simulink model "FinalProject"  (R2025b)
settings: Solver=ode3  StartTime=0.0  StopTime=1  RelTol=1e-3
libraries: spsMosfetLib x12, simulink x9, spsDCVoltageSourceLib x4, spsCurrentMeasurementLib x1, spsSeriesRLCBranchLib x1, spsVoltageMeasurementLib x1, sps_lib x1
settings Model: Creator=RGUKT  LastModifiedBy=RGUKT

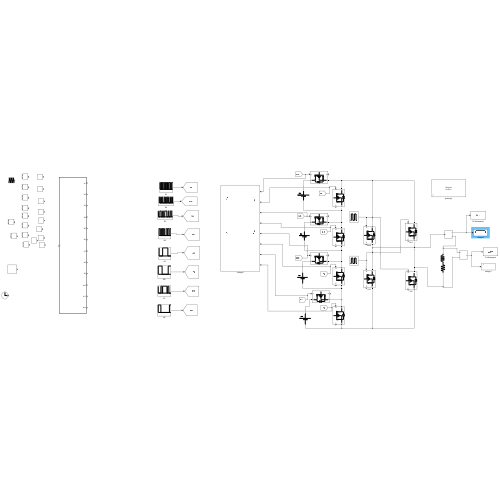
[thumbnail: Simulink's stored preview of the top-level diagram]
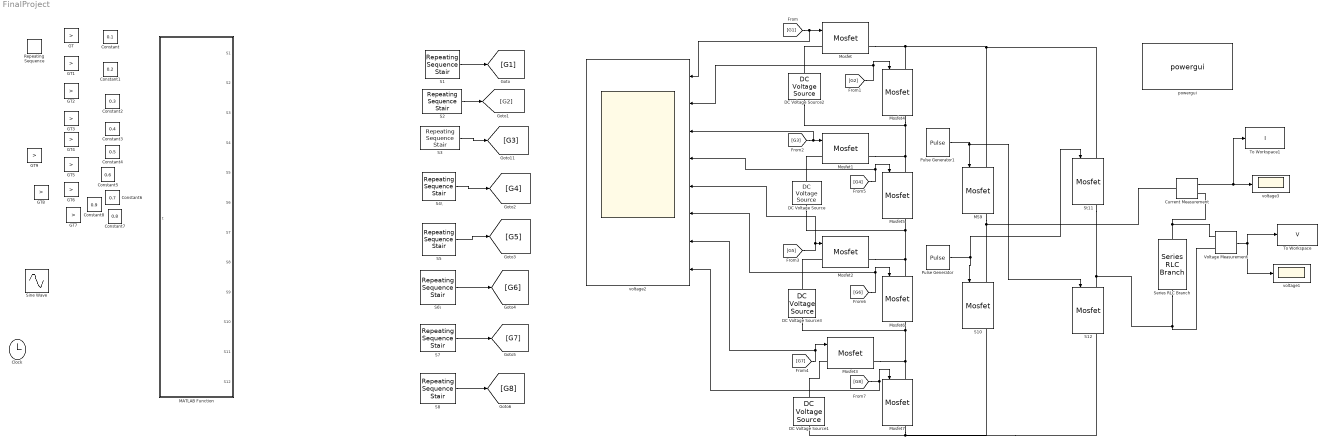
== system FinalProject ==
  Clock : Clock
  Constant : Constant  Value=0.1
  Constant1 : Constant  Value=0.2
  Constant2 : Constant  Value=0.3
  Constant3 : Constant  Value=0.4
  Constant4 : Constant  Value=0.5
  Constant5 : Constant  Value=0.6
  Constant6 : Constant  Value=0.7
  Constant7 : Constant  Value=0.8
  Constant8 : Constant  Value=0.9
  Current Measurement : spsCurrentMeasurementLib/Current Measurement  PhasorSimulation=off  OutputType=Complex  PSBequivalent=0
  DC Voltage Source : spsDCVoltageSourceLib/DC Voltage Source  Amplitude=20  Measurements=None
  DC Voltage Source1 : spsDCVoltageSourceLib/DC Voltage Source  Amplitude=40  Measurements=None
  DC Voltage Source2 : spsDCVoltageSourceLib/DC Voltage Source  Amplitude=10  Measurements=None
  DC Voltage Source3 : spsDCVoltageSourceLib/DC Voltage Source  Amplitude=30  Measurements=None
  GT{,1..9} (10 alike) : RelationalOperator  Operator=>  OutDataTypeStr=boolean  RndMeth=Simplest  InputSameDT=off
  MATLAB Function : MATLAB Function  TreatAsAtomicUnit=on
  MS9 : spsMosfetLib/Mosfet  Ron=0.1  Lon=0  Rd=0.01  Vfd=0  IC=0  Rs=1e5  Cs=inf  Measurements=on
  Mosfet{,1..7} (8 alike) : spsMosfetLib/Mosfet  Ron=0.1  Lon=0  Rd=0.01  Vfd=0  IC=0  Rs=1e5  Cs=inf  Measurements=on
  Pulse Generator : DiscretePulseGenerator  PulseType=Time based  Period=0.02  PulseWidth=50  PhaseDelay=0.01
  Pulse Generator1 : DiscretePulseGenerator  PulseType=Time based  Period=0.02  PulseWidth=50
  Repeating Sequence : simulink/Sources/Repeating Sequence  rep_seq_t=[0 0.01 0.02]  rep_seq_y=[0 1 0]
  S1 : simulink/Sources/Repeating Sequence Stair  OutValues=[0 1 0 1 0 1 1 0 1 0 1 0 1 0 1 1 0 1 0 1].'  tsamp=0.0005  OutMin=[]  OutMax=[]  OutDataTypeStr=double  OutputDataTypeScalingMode=double  OutDataType=fixdt(0,8)  ConRadixGroup=Best Precision: Vector-wise  OutScaling=2^-12
  S10 : spsMosfetLib/Mosfet  Ron=0.1  Lon=0  Rd=0.01  Vfd=0  IC=0  Rs=1e5  Cs=inf  Measurements=on
  S12 : spsMosfetLib/Mosfet  Ron=0.1  Lon=0  Rd=0.01  Vfd=0  IC=0  Rs=1e5  Cs=inf  Measurements=on
  S2 : simulink/Sources/Repeating Sequence Stair  OutValues=[1 0 1 0 1 0 0 1 0 1 0 1 0 1 0 0 1 0 1 0].'  tsamp=0.0005  OutMin=[]  OutMax=[]  OutDataTypeStr=double  OutputDataTypeScalingMode=double  OutDataType=fixdt(0,8)  ConRadixGroup=Best Precision: Vector-wise  OutScaling=2^-12
  S3 : simulink/Sources/Repeating Sequence Stair  OutValues=[0 0 1 1 0 0 1 0 0 1 1 1 0 0 1 0 0 1 1 0].'  tsamp=0.0005  OutMin=[]  OutMax=[]  OutDataTypeStr=double  OutputDataTypeScalingMode=double  OutDataType=fixdt(0,8)  ConRadixGroup=Best Precision: Vector-wise  OutScaling=2^-12
  S4\ : simulink/Sources/Repeating Sequence Stair  OutValues=[1 1 0 0 1 1 0 1 1 0 0 0 1 1 0 1 1 0 0 1].'  tsamp=0.0005  OutMin=[]  OutMax=[]  OutDataTypeStr=double  OutputDataTypeScalingMode=double  OutDataType=fixdt(0,8)  ConRadixGroup=Best Precision: Vector-wise  OutScaling=2^-12
  S5 : simulink/Sources/Repeating Sequence Stair  OutValues=[0 0 0 0 0 0 1 1 1 1 1 1 1 1 1 0 0 0 0 0].'  tsamp=0.0005  OutMin=[]  OutMax=[]  OutDataTypeStr=double  OutputDataTypeScalingMode=double  OutDataType=fixdt(0,8)  ConRadixGroup=Best Precision: Vector-wise  OutScaling=2^-12
  S6\ : simulink/Sources/Repeating Sequence Stair  OutValues=[1 1 1 1 1 1 0 0 0 0 0 0 0 0 0 0 1 1 1 1].'  tsamp=0.0005  OutMin=[]  OutMax=[]  OutDataTypeStr=double  OutputDataTypeScalingMode=double  OutDataType=fixdt(0,8)  ConRadixGroup=Best Precision: Vector-wise  OutScaling=2^-12
  S7 : simulink/Sources/Repeating Sequence Stair  OutValues=[0 0 0 0 1 1 0 1 1 1 1 1 1 1 0 1 1 0 0 0].'  tsamp=0.0005  OutMin=[]  OutMax=[]  OutDataTypeStr=double  OutputDataTypeScalingMode=double  OutDataType=fixdt(0,8)  ConRadixGroup=Best Precision: Vector-wise  OutScaling=2^-12
  S8 : simulink/Sources/Repeating Sequence Stair  OutValues=[1 1 1 1 0 0 0 0 0 0 0 0 0 0 0 0 0 0 1 1].'  tsamp=0.0005  OutMin=[]  OutMax=[]  OutDataTypeStr=double  OutputDataTypeScalingMode=double  OutDataType=fixdt(0,8)  ConRadixGroup=Best Precision: Vector-wise  OutScaling=2^-12
  Series RLC Branch : spsSeriesRLCBranchLib/Series RLC Branch  LConnTagsString=__new0  RConnTagsString=__new0  BranchType=RL  Resistance=10  Inductance=0.007  SetiL0=off  InitialCurrent=0  Capacitance=1e-6  Setx0=off  InitialVoltage=0  Measurements=None
  Sine Wave : Sin  Frequency=314.15  SampleTime=0
  St11 : spsMosfetLib/Mosfet  Ron=0.1  Lon=0  Rd=0.01  Vfd=0  IC=0  Rs=1e5  Cs=inf  Measurements=on
  To Workspace : ToWorkspace  VariableName=V  SaveFormat=Structure With Time  SampleTime=-1
      settings: Save2DSignal=2-D array (concatenate along first dimension)
  To Workspace1 : ToWorkspace  VariableName=I  SaveFormat=Structure With Time  SampleTime=-1
      settings: Save2DSignal=2-D array (concatenate along first dimension)
  Voltage Measurement : spsVoltageMeasurementLib/Voltage Measurement  PhasorSimulation=off  OutputType=Complex  PSBequivalent=0
  powergui : sps_lib/powergui  Priority=1  SimulationMode=Discrete  SampleTime=5e-06  frequency=60  Iterations=50  frequencyindice=0  Pbase=100e6  ErrMax=1e-4  UnitsV=kV  UnitsW=MW  buscounter=0  FunctionMessages=off  echomessages=off  EnableUseOfTLC=off  CurrentSourceSwitches=off  DisableSnubberDevices=off  DisableRonSwitches=off  DisableVfSwitches=off  DisplayEquations=off  AutomaticDiscreteSolvers=off  SolverType=Tustin/Backward Euler (TBE)  Interpol=off  ExternalGateDelay=off  methode=off  Ts=100  x0status=blocks  SPID=on  SwTol=0  HookPort=off  NonlinearTolerance=1e-4  nMaxIteration=100  ContinueOnMaxIteration=off  RestoreLinks=warning  ResistiveCurrentMeasurement=off  Frange=[0:2:500]  Ylog=off  Xlog=on  ShowGrid=off  save=off  variable=ZData  structure=0  ZoomFFT=off  StartTime=0.0  cycles=1  DisplayStyle=1  fundamental=60  FreqAxis=off  MaxFrequency=1000  frequencyindicesteady=1  RmsSteady=1  display=off
  voltage1 : Scope
      settings: ActiveDisplayYMinimum=-117.92329789248066  ActiveDisplayYMaximum=117.9232978938367
  voltage2 : Scope  NumInputPorts=8
      settings: ActiveDisplayYMinimum=-0.12499999999999997  ActiveDisplayYMaximum=1.125  DataLoggingVariableName=ScopeData2
  voltage3 : Scope
      settings: ActiveDisplayYMinimum=-11.792329789248956  ActiveDisplayYMaximum=11.7923297893823
  wires:
  Voltage Measurement/1 -> To Workspace/1, voltage1/1
  S8/1 -> [G8]
  S7/1 -> [G7]
  S6\/1 -> [G6]
  S5/1 -> [G5]
  S4\/1 -> [G4]
  [G1] -> voltage2/1, Mosfet/1
  [G3] -> voltage2/3, Mosfet1/1
  [G5] -> voltage2/5, Mosfet2/1
  [G7] -> voltage2/7, Mosfet3/1
  [G2] -> voltage2/2, Mosfet4/1
  [G4] -> voltage2/4, Mosfet5/1
  [G6] -> voltage2/6, Mosfet6/1
  [G8] -> voltage2/8, Mosfet7/1
  S1/1 -> [G1]
  S2/1 -> [G2]
  S3/1 -> [G3]
  Pulse Generator1/1 -> S12/1, MS9/1
  Pulse Generator/1 -> S10/1, St11/1
  Current Measurement/1 -> To Workspace1/1, voltage3/1
  connections:
  DC Voltage Source2/RConn1 -- Mosfet/LConn1
  Mosfet4/LConn1 -- St11/LConn1 -- MS9/LConn1 -- Mosfet/RConn1
  DC Voltage Source/RConn1 -- Mosfet1/LConn1
  DC Voltage Source3/RConn1 -- Mosfet2/LConn1
  DC Voltage Source1/RConn1 -- Mosfet3/LConn1
  S12/RConn1 -- S10/RConn1 -- DC Voltage Source1/LConn1 -- Mosfet7/RConn1
  Mosfet4/RConn1 -- Mosfet5/LConn1 -- Mosfet1/RConn1 -- DC Voltage Source2/LConn1
  Mosfet6/LConn1 -- Mosfet2/RConn1 -- DC Voltage Source/LConn1 -- Mosfet5/RConn1
  Mosfet7/LConn1 -- Mosfet3/RConn1 -- DC Voltage Source3/LConn1 -- Mosfet6/RConn1
  Series RLC Branch/LConn1 -- St11/RConn1 -- S12/LConn1 -- Voltage Measurement/LConn2
  Series RLC Branch/RConn1 -- Current Measurement/RConn1 -- Voltage Measurement/LConn1
  MS9/RConn1 -- Current Measurement/LConn1 -- S10/LConn1

== matlab function FinalProject/MATLAB Function ==
  data: t input; S1 output; S2 output; S3 output; S4 output; S5 output; S6 output; S7 output; S8 output; S9 output; S10 output; S11 output; S12 output
function [S1,S2,S3,S4,S5,S6,S7,S8,S9,S10,S11,S12] = fcn(t)

f = 50;
w = 2*pi*f;

% Sine reference
Vref = sin(w*t);

% 10 levels (normalized)
levels = [-1 -0.9 -0.8 -0.7 -0.6 -0.5 -0.4 -0.3 -0.2 -0.1 ...
           0 ...
          0.1 0.2 0.3 0.4 0.5 0.6 0.7 0.8 0.9 1];

% Find nearest level
[~, idx] = min(abs(Vref - levels));
L = levels(idx);

% Convert to integer level (0 to 10)
L = round(L * 10);

% Initialize switches
S1=0; S2=0; S3=0; S4=0;
S5=0; S6=0; S7=0; S8=0;
S9=0; S10=0; S11=0; S12=0;

% Polarity
if L >= 0
    S9=1; S10=1;
else
    S11=1; S12=1;
end

L = abs(L);

% Switching table (same as paper)
switch L
    
    case 0
        S2=1; S4=1; S6=1; S8=1;

    case 1
        S1=1; S4=1; S6=1; S8=1;

    case 2
        S2=1; S3=1; S6=1; S8=1;

    case 3
        S1=1; S3=1; S6=1; S8=1;

    case 4
        S1=1; S4=1; S6=1; S7=1;

    case 5
        S1=1; S4=1; S5=1; S7=1;

    case 6
        S1=1; S3=1; S5=1; S8=1;

    case 7
        S2=1; S4=1; S5=1; S7=1;

    case 8
        S1=1; S4=1; S5=1; S7=1;

    case 9
        S2=1; S3=1; S5=1; S7=1;

    case 10
        S1=1; S3=1; S5=1; S7=1;

end
